simulink model "BEST2020_gamepad_template"  (R2020a)
settings: Solver=ode23t  StartTime=0.0  StopTime=180.1  FixedStep=0.05  RelTol=1e-3  EnableMultiTasking=on
model workspace (MAT data in the model file):
  mapForSim.obsMap = [0 0 0 0 0 0 0 0 0 0 0 0 ... (4194304 elements, 2048x2048)]
  mapForSim.scaleFactor = 409.6
  mapForSim.simMap = robotics.BinaryOccupancyGrid
  mapForSim.simMap.Grid = [1 1 1 1 1 1 1 1 1 1 1 1 ... (4194304 elements, 2048x2048)]
  mapForSim.simMap.LayerName = "binaryLayer"
  mapForSim.simMap.Index = matlabshared.autonomous.internal.CircularBufferIndex
  mapForSim.simMap.Index.Head = [1 1]
  mapForSim.simMap.Index.Size = [2048 2048]
  mapForSim.simMap.Index.NewRegions = [0 0 0 0]
  mapForSim.simMap.Index.DropEntireMap = 0
  mapForSim.simMap.Index.DropTwoRegions = [0 0]
  mapForSim.simMap.Buffer = matlabshared.autonomous.internal.CircularBuffer
  mapForSim.simMap.Buffer.ConstVal = 0
  mapForSim.simMap.Buffer.DataType = 'logical'
  mapForSim.simMap.Buffer.Index = matlabshared.autonomous.internal.CircularBufferIndex
  mapForSim.simMap.Buffer.Index.Head = [1 1]
  mapForSim.simMap.Buffer.Index.Size = [2048 2048]
  mapForSim.simMap.Buffer.Index.NewRegions = [0 0 0 0]
  mapForSim.simMap.Buffer.Index.DropEntireMap = 0
  mapForSim.simMap.Buffer.Index.DropTwoRegions = [0 0]
  mapForSim.simMap.Buffer.Buffer = [1 1 1 1 1 1 1 1 1 1 1 1 ... (4194304 elements, 2048x2048)]
  mapForSim.simMap.DefaultValueInternal = 0
  mapForSim.simMap.HasParent = 0
  mapForSim.simMap.Resolution = 409.6
  mapForSim.simMap.GridSize = [2048 2048]
  mapForSim.simMap.GridOriginInLocal = [0 0]
  mapForSim.simMap.LocalOriginInWorld = [0 0]
  mapForSim.simMap.Width = 5
  mapForSim.simMap.Height = 5
  mapForSim.simMap.LocalOriginInWorldInternal = [0 0]
  occGrid = robotics.BinaryOccupancyGrid
  occGrid.Grid = [1 1 1 1 1 1 1 1 1 1 1 1 ... (4194304 elements, 2048x2048)]
  occGrid.LayerName = "binaryLayer"
  occGrid.Index = matlabshared.autonomous.internal.CircularBufferIndex
  occGrid.Index.Head = [1 1]
  occGrid.Index.Size = [2048 2048]
  occGrid.Index.NewRegions = [0 0 0 0]
  occGrid.Index.DropEntireMap = 0
  occGrid.Index.DropTwoRegions = [0 0]
  occGrid.Buffer = matlabshared.autonomous.internal.CircularBuffer
  occGrid.Buffer.ConstVal = 0
  occGrid.Buffer.DataType = 'logical'
  occGrid.Buffer.Index = matlabshared.autonomous.internal.CircularBufferIndex
  occGrid.Buffer.Index.Head = [1 1]
  occGrid.Buffer.Index.Size = [2048 2048]
  occGrid.Buffer.Index.NewRegions = [0 0 0 0]
  occGrid.Buffer.Index.DropEntireMap = 0
  occGrid.Buffer.Index.DropTwoRegions = [0 0]
  occGrid.Buffer.Buffer = [1 1 1 1 1 1 1 1 1 1 1 1 ... (4194304 elements, 2048x2048)]
  occGrid.DefaultValueInternal = 0
  occGrid.HasParent = 0
  occGrid.Resolution = 409.6
  occGrid.GridSize = [2048 2048]
  occGrid.GridOriginInLocal = [0 0]
  occGrid.LocalOriginInWorld = [0 0]
  occGrid.Width = 5
  occGrid.Height = 5
  occGrid.LocalOriginInWorldInternal = [0 0]
undefined symbols (not defined in the file): cellLevel, cellPose, cellTypeArray, FloorSurface, isoPoses, platformPoses, PlowSurface, Ref, RobotSurface, WallSurface, X, Y, Z
libraries: sm_lib x286, nesl_utility x157, simulink x72, vexcommonlib x2, vrlib x1
(part 1 of 14)
settings Model: EnablePacing=on  ExtModeTrigDuration=25  Creator=scastro  LastModifiedBy=Hashim Aziz
settings SolverCC: AlgebraicLoopSolver=LineSearch
settings DataIOCC: LimitDataPoints=on  ReturnWorkspaceOutputs=off
settings OptimizationCC: DefaultParameterBehavior=Inlined  PassReuseOutputArgsAs=Individual arguments  MaxStackSize=64  EfficientTunableParamExpr=on
settings DebuggingCC: ParameterPrecisionLossMsg=none  ParameterTunabilityLossMsg=error  UnconnectedLineMsg=none  AllowSymbolicDim=off  SFUnexpectedBacktrackingDiag=warning  SFNoUnconditionalDefaultTransitionDiag=warning  SFExecutionAtInitializationDiag=none  ArithmeticOperatorsInVariantConditions=warning
settings HardwareCC: ProdBitPerPointer=32  ProdBitPerSizeT=32  ProdBitPerPtrDiffT=32  ProdLargestAtomicInteger=Long  ProdLargestAtomicFloat=Double  ProdWordSize=32  ProdHWDeviceType=ARM Compatible->ARM Cortex
settings SFSimCC: SimUseLocalCustomCode=off  MATLABDynamicMemAlloc=off  CustomCodeUndefinedFunction=UseInterfaceOnly
settings RTWCC: SystemTargetFile=ert.tlc  TemplateMakefile=ert_default_tmf  GenerateReport=on  RTWUseLocalCustomCode=off  Toolchain=GNU Tools for ARM Embedded Processors  IncludeHyperlinkInReport=on  LaunchReport=on  GenerateTraceInfo=on  GenerateTraceReport=on  GenerateTraceReportSl=on  GenerateTraceReportSf=on  GenerateTraceReportEml=on
settings CodeAppCC: ForceParamTrailComments=on  IgnoreCustomStorageClasses=off  OperatorAnnotations=on  SimulinkDataObjDesc=on  SFDataObjDesc=on  InsertBlockDesc=on
settings ERTTargetCC: ExtModeStaticAllocSize=2048  ERTCustomFileTemplate=example_file_process.tlc
settings ConfigComp: CovMetricSettings=dw  CovHtmlReporting=on  CovSaveCumulativeToWorkspaceVar=on  CovSaveSingleToWorkspaceVar=on  CovExternalEMLEnable=off  CovSFcnEnable=off
settings SimscapeCC: SimscapeNominalValues="[{\"value\":\"10\",\"unit\":\"V\"},{\"value\":\"1\",\"unit\":\"A\"},{\"value\":\"10\",\"unit\":\"N*m\"},{\"value\":\"10\",\"unit\":\"bar\"},{\"value\":\"100\",\"unit\":\"kJ/kg\"},{\"value\":\"1\",\"unit\":\"kW\"},{\"value\":\"300\",\"unit\":\"K\"},{\"value\":\"100\",\"unit\":\"cm^3/s\"},{\"value\":\"1\",\"unit\":\"kN\"},{\"value\":\"1\",\"unit\":\"g/cm^3\"},{\"value\":\"1\",\"unit\":\"l\"},{\"value\":\"1\",\"unit\":\"cm^2\"},{\"value\":\"60\",\"unit\":\"Hz\"}]"  SimscapeLogOpenViewer=on  SimscapeLogDataHistory=10000
settings ConfigurationSet: Description=SimMechanics 2G
settings DiagnosticsConfigSet: SimMechanicsRigidlyBoundBlock=none
settings ExplorerConfigSet: InternalSimMechanicsExplorerSettings="<ExplorerConfiguration><canonicalview>default</canonicalview><AnimationSetting><BasePlaybackSpeed>1.0</BasePlaybackSpeed><PlaybackSpeedFactor>1.0</PlaybackSpeedFactor></AnimationSetting><TilePanel><TileInfo><Tiles Columns=\"2\" Count=\"3\" Rows=\"2\"><Column Weight=\"0.5\"/><Column Weight=\"0.5\"/><Row Weight=\"0.668\"/><Row Weight=\"0.332\"/><Tile Height=\"1\" Width=\"2\" X=\"0\" Y=\"0\"/><Tile Height=\"1\" Width=\"1\" X=\"0\" Y=\"1\"/><Tile Height=\"1\" Width=\"1\" X=\"1\" Y=\"1\"/></Tiles></TileInfo><SceneInfo><SceneViewer><BGColor><R>0.60000002384185791</R><G>0.60000002384185791</G><B>0.60000002384185791</B></BGColor><Camera><DoPerspective>off</DoPerspective><Position><X>2.41066835351507569</X><Y>-4.14908984137515624</Y><Z>3.70193270331160607</Z></Position><Center><X>1.01728519569986009</X><Y>-1.70616544620136401</Y><Z>1.53735654734938021</Z></Center><Up><X>-0.394111566140174063</X><Y>0.473277490849461246</Y><Z>0.787835319143396218</Z></Up><ViewLimDist>1</ViewLimDist><YLim>1.30936523991048004</YLim><XLim>3.19500799558994419</XLim></Camera></SceneViewer><SceneViewer><BGColor><R>0.60000002384185791</R><G>0.60000002384185791</G><B>0.60000002384185791</B></BGColor><Camera><DoPerspective>on</DoPerspective><Position><X>-2.5</X><Y>0</Y><Z>0.469999999999999973</Z></Position><Center><X>-1.56030737921409157</X><Y>0</Y><Z>0.12797985667433126</Z></Center><Up><X>0.342020143325668713</X><Y>0</Y><Z>0.939692620785908428</Z></Up><ViewLimDist>1</ViewLimDist><YLim>0.466307658154998583</YLim><XLim>1.15289562108260379</XLim></Camera></SceneViewer><SceneViewer><BGColor><R>0.60000002384185791</R><G>0.60000002384185791</G><B>0.60000002384185791</B></BGColor><Camera><DoPerspective>off</DoPerspective><Position><X>-0.165662310308284766</X><Y>-0.309058030467383449</Y><Z>7.45210262533490209</Z></Position><Center><X>-0.165662310308284766</X><Y>-0.309058030467383449</Y><Z>0.069999846435872648</Z></Center><Up><X>0</X><Y>1</Y><Z>-0</Z></Up><ViewLimDist>1</ViewLimDist><YLim>2.10368262272791195</YLim><XLim>5.20112942919845711</XLim></Camera></SceneViewer></SceneInfo></TilePanel><MechEditorPanel><Cameras><Camera><Id>Camera1</Id><Value><Name>RobotView</Name><NativeCamera><PositionTrackingFeature>BEST_Robotics_2020_Game_Double_Click.BEST_2020_Robot.Body.RobotCamera.F</PositionTrackingFeature><CenterTrackingFeature>BEST_Robotics_2020_Game_Double_Click.BEST_2020_Robot.Body.RobotCamera.F</CenterTrackingFeature><UpVectorTrackingFeature>BEST_Robotics_2020_Game_Double_Click.BEST_2020_Robot.Body.RobotCamera.F</UpVectorTrackingFeature><CenterTrackingOrigin>off</CenterTrackingOrigin><CenterTrackingDirection>+X</CenterTrackingDirection><UpVectorTrackingDirection>+Z</UpVectorTrackingDirection></NativeCamera></Value></Camera></Cameras><GfxPanelCameraMap><MapElement CameraMLId=\"Camera1\" GfxPanelIndex=\"1\"/></GfxPanelCameraMap><VideoCreator><PlaybackSpeedRatio>1.0</PlaybackSpeedRatio><FrameRate>30</FrameRate><VideoFormat>Motion JPEG AVI</VideoFormat><FrameSize>auto</FrameSize></VideoCreator></MechEditorPanel></ExplorerConfiguration>"

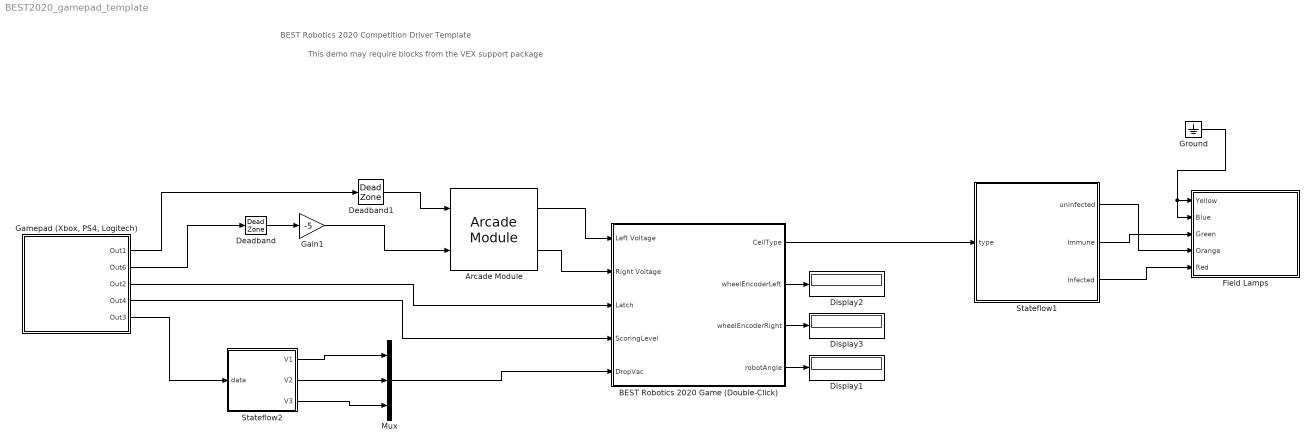
== system BEST2020_gamepad_template ==
  note: BEST Robotics 2020 Competition Driver Template
  note: This demo may require blocks from the VEX support package
  Arcade Module : vexcommonlib/Arcade Module  BlockPlatform=vexarmcortex
      settings: SourceProductBaseCode=EC_VEX_MICRO,VEXV5
  BEST Robotics 2020 Game (Double-Click) : Subsystem  mask(RP BEST Robotics 2020 Challenge){gameTime=180, field=Random, rvis=on, sensor=off, autoField=off, wheelBase=0.5, wheelRadius=0.1, robotColor=[0.5 0 0], wheelThickness=0.025, chassisThickness=0.05, wheelMass=1, chassisMass=1.5}
      mask prompts: gameTime "Game Time (s)"; field "Field Layout"; rvis "Show cell type after run (Runs slower)"; sensor "Activate Gripper Sensor (Not allowed during competition)"; autoField "Autonomous Configuration"; wheelBase "Distance between wheels [m]"; wheelRadius "Wheel radius [m]"; robotColor "Color [R G B]"; wheelThickness "Wheel Thickness [m]"; chassisThickness "Chassis Thickness [m]"; wheelMass "Wheel Mass [kg]"; chassisMass "Chassis Mass [kg]"
      mask help:
      | This block contains a virtual game for the BEST Robotics 2020 competition. Please refere to the instructions provided by competition organizers for more information on game rules.
      |
      | Inputs:
      | Motor Voltages (Torque) [-127 to 127]
      | LatchCell (Pickup Cell) [0 or 1]
      | ScoringLevel (Floor or Platform) [0 or 1]
      | DropVac (Release vaccine) [0 or 1] Array of 3
      |
      | Outputs:
      | Cell Type (Uninfected, Immune, Infected) [0 ,1 or 2]
      | Sensors (See inside block for sensor properties and outputs)
      |
      | For MATLAB and Simulink related questions please email: roboticsarena@mathworks.com
      mask init:
      | autochoice=get_param(gcb,'autoField');
      | choice=get_param(gcb,'field');
      | time=get_param(gcb,'gameTime');
      | set_param(gcs,'StopTime',num2str(str2num(time)+0.1));
      | 
      | if strcmp(choice,'Practice 1')
      |   BEST2020GameConfig1 
      | elseif strcmp(choice,'Practice 2')
      |   BEST2020GameConfig2 
      | elseif strcmp(choice,'Practice 3')
      |   BEST2020GameConfig3 
      | elseif strcmp(choice,'Random')
      |   BEST2020GameConfigRand
      | elseif strcmp(autochoice,"on")
      |    if strcmp(choice,'Competition 1 (Provided during competition)')
      |      BEST2020GameConfigAuto1
      |    elseif strcmp(choice,'Competition 2 (Provided during competition)')
      |      BEST2020GameConfigAuto2
      |    elseif strcmp(choice,'Competition 3 (Provided during competition)')
      |      BEST2020GameConfigAuto3
      |    elseif strcmp(choice,'Competition 4 (Provided during competition)')
      |      BEST2020GameConfigAuto4
      |    elseif strcmp(choice,'Competition 5 (Provided during competition)')
      |      BEST2020GameConfigAuto5
      |    elseif strcmp(choice,'Competition 6 (Provided during competition)')
      |      BEST2020GameConfigAuto6
      |    elseif strcmp(choice,'Competition 7 (Provided during competition)')
      |      BEST2020GameConfigAuto7
      |    elseif strcmp(choice,'Competition 8 (Provided during competition)')
      |      BEST2020GameConfigAuto8
      |    else
      |      BEST2020GameConfigAuto1
      |    end
      | elseif strcmp(choice,'Competition 1 (Provided during competition)')
      |   BEST2020GameConfigComp1
      | elseif strcmp(choice,'Competition 2 (Provided during competition)')
      |   BEST2020GameConfigComp2
      | elseif strcmp(choice,'Competition 3 (Provided during competition)')
      |   BEST2020GameConfigComp3
      | elseif strcmp(choice,'Competition 4 (Provided during competition)')
      |   BEST2020GameConfigComp4
      | elseif strcmp(choice,'Competition 5 (Provided during competition)')
      |   BEST2020GameConfigComp5
      | elseif strcmp(choice,'Competition 6 (Provided during competition)')
      |   BEST2020GameConfigComp6
      | elseif strcmp(choice,'Competition 7 (Provided during competition)')
      |   BEST2020GameConfigComp7
      | elseif strcmp(choice,'Competition 8 (Provided during competition)')
      |   BEST2020GameConfigComp8
      | else
      |   BEST2020GameConfig1 
      | end
      mask TypeOptions field: Practice 1 | Practice 2 | Practice 3 | Random | Competition 1 (Provided during competition) | Competition 2 (Provided during competition) | Competition 3 (Provided during competition) | Competition 4 (Provided during competition) | Competition 5 (Provided during competition) | Competition 6 (Provided during competition) | Competition 7 (Provided during competition) | Competition 8 (Provided during competition)
      mask Callback rvis:
      | visual=get_param(gcb,'rvis');
      | for i=1:21
      |     if strcmp(visual,'off')
      |         set_param([gcb '/Cells/Object' num2str(i) '/EndVisuals'],'Commented','on');
      |     else
      |         set_param([gcb '/Cells/Object' num2str(i) '/EndVisuals'],'Commented','off');
      |     end
      | end
      mask TypeOptions wheelThickness: BEST 2020 Robot/wheelThickness
      mask TypeOptions chassisThickness: BEST 2020 Robot/chassisThickness
      mask TypeOptions wheelMass: BEST 2020 Robot/wheelMass
      mask TypeOptions chassisMass: BEST 2020 Robot/chassisMass
      mask DialogControl Container8 Prompt: Game Settings
      mask DialogControl Container4 Prompt: Robot settings
      mask Display:
      | image('BEST2020Environment.png')
      | port_label('input',1,'RightMotor')
      | port_label('input',2,'LeftMotor')
      | port_label('input',3,'LatchCell')
      | port_label('input',4,'ScoringLevel')
      | port_label('input',5,'DropVac')
      | port_label('output',1,'CellType')
      | port_label('output',2,'LeftEncoder')
      | port_label('output',3,'RightEncoder')
      | port_label('output',4,'RobotAngle')
  Deadband : DeadZone  SaturateOnIntegerOverflow=on
  Deadband1 : DeadZone  SaturateOnIntegerOverflow=on
  Display1 : Display
  Display2 : Display
  Display3 : Display
  Field Lamps : Subsystem
      mask Display:
      | image('lamps.PNG')
      | port_label('input',1,'Yellow')
      | port_label('input',2,'Blue')
      | port_label('input',3,'Green')
      | port_label('input',4,'Orange')
      | port_label('input',5,'Red')
  Gain1 : Gain  Gain=-5
  "Gamepad (Xbox, PS4, Logitech)" : Subsystem
      mask Display:
      | pic = imread(fullfile(codertarget.vexcommon.internal.getRootDir(),'resources','Gamepad_Controller.png'));
      | image(pic);
  Ground : Ground
  Mux : Mux  Inputs=3
  Stateflow1 : Stateflow chart  AncestorBlock=RoboticsPlayground/Utilities and Hardware/Stateflow  TreatAsAtomicUnit=on
  Stateflow2 : Stateflow chart  AncestorBlock=RoboticsPlayground/Utilities and Hardware/Stateflow  TreatAsAtomicUnit=on
  wires:
  Mux/1 -> BEST Robotics 2020 Game (Double-Click)/5(DropVac)
  BEST Robotics 2020 Game (Double-Click)/1(CellType) -> Stateflow1/1(type)
  BEST Robotics 2020 Game (Double-Click)/4(robotAngle) -> Display1/1
  BEST Robotics 2020 Game (Double-Click)/3(wheelEncoderRight) -> Display3/1
  BEST Robotics 2020 Game (Double-Click)/2(wheelEncoderLeft) -> Display2/1
  Arcade Module/1 -> BEST Robotics 2020 Game (Double-Click)/1(Left Voltage)
  Arcade Module/2 -> BEST Robotics 2020 Game (Double-Click)/2(Right Voltage)
  Gain1/1 -> Arcade Module/2
  Deadband/1 -> Gain1/1
  Deadband1/1 -> Arcade Module/1
  "Gamepad (Xbox, PS4, Logitech)"/4(Out4) -> BEST Robotics 2020 Game (Double-Click)/4(ScoringLevel)
  Stateflow1/3(Infected) -> Field Lamps/5(Red)
  Stateflow1/2(Immune) -> Field Lamps/3(Green)
  Stateflow1/1(uninfected) -> Field Lamps/4(Orange)
  Ground/1 -> Field Lamps/2(Blue), Field Lamps/1(Yellow)
  Stateflow2/1(V1) -> Mux/1
  Stateflow2/2(V2) -> Mux/2
  Stateflow2/3(V3) -> Mux/3
  "Gamepad (Xbox, PS4, Logitech)"/5(Out3) -> Stateflow2/1(data)
  "Gamepad (Xbox, PS4, Logitech)"/1(Out1) -> Deadband1/1
  "Gamepad (Xbox, PS4, Logitech)"/2(Out6) -> Deadband/1
  "Gamepad (Xbox, PS4, Logitech)"/3(Out2) -> BEST Robotics 2020 Game (Double-Click)/3(Latch)

== system BEST2020_gamepad_template/BEST Robotics 2020 Game (Double-Click) ==
  note: DO NOT CHANGE THIS MODEL!
  Left Voltage : Inport
  Right Voltage : Inport  Port=2
  Latch : Inport  Port=3
  ScoringLevel : Inport  Port=4
  DropVac : Inport  Port=5
  Arena : Subsystem  mask(RP Grid Arena){length=7, width=7}
      mask prompts: length "Arena length [m]"; width "Arena width [m]"
      mask help: This block is an arena for robots to operate within. This arena implements contact between one robot and the walls and also introduces a floor grid for better visualization. Connect to other robots within the library using the corresponding "Robot" and "Ref" ports.
      mask DialogControl Container5 Prompt: Arena dimensions
      mask Display:
      | image('BEST2020Arena.png')
      | port_label('Lconn',1,'RP-Bus')
  BEST 2020 Robot : Subsystem  mask(RP Contact Tank Robot){robotId=1, wheelRadius=wheelRadius, wheelBase=wheelBase, wheelThickness=wheelThickness, chassisThickness=chassisThickness, startPose=[-2 0], choice=off, sensorTs=0.05, wheelMass=wheelMass, chassisMass=chassisMass, maxWheelTorque=2, wheelColor=[0.25 0.25 0.25], chassisColor=robotColor}
      mask prompts: robotId "Robot ID"; wheelRadius "Wheel Radius [m]"; wheelBase "Wheelbase [m]"; wheelThickness "Wheel Thickness [m]"; chassisThickness "Chassis Thickness [m]"; startPose "Start Position [m]"; choice "Reverse Start Position"; sensorTs "Sensor sample time [s]"; wheelMass "Wheel Mass [kg]"; chassisMass "Chassis Mass [kg]"; maxWheelTorque "Maximum wheel torque [N*m]"; wheelColor "Wheel Color"; chassisColor "Chassis Color"
      mask help:
      | This robot implements contact between the robot wheels and the floor of an arena. The stck-slip friction implemented using contact force libraries makes the robot behavior more realistic. The inputs to the robot are now motor torque, which is set using the Robotics Playground Motor blocks. The motor mappings are as follows:
      |
      | Motor 1 -> Left wheel motor torque
      | Motor 2 -> Right wheel motor torque
      mask DialogControl KinContainer Prompt: Kinematics
      mask DialogControl DynamicsContainer Prompt: Dynamics
      mask DialogControl AppearanceContainer Prompt: Appearance
      mask Display:
      | image('BEST2020Robot.png')
      | port_label('Rconn',1,'RP-Bus')
  Cells : Subsystem
      mask Display: image('BEST2020Cells.png')
  Compass Sensor : Subsystem  mask(RP Compass Sensor){sensorTs=0.1}
      mask prompts: sensorTs "Sensor sample time [s]"
      mask help: This sensor outputs the rotation in degrees as measured from the robot center relative to the world coordinate frame.
      mask Help: web('compass_sensor.htm')
      mask DialogControl senCont Prompt: Sensor Characteristics
      mask Display:
      | color('white');
      | plot([100,100,100,100]*1,[100,100,100,100]*1);
      | plot([100,100,100,100]*0,[100,100,100,100]*0);
      | image('Compass.png','center')
      | color('blue');
  Game Control : Subsystem
  Left Encoder : Subsystem  mask(RP Motor Encoder){rstChoice=No reset, ticks=180, detectDir=off, sensorTs=0.1}
      mask prompts: rstChoice "Reset option"; ticks "Ticks per rotation"; detectDir "Detect direction of rotation"; sensorTs "Sensor sample time [s]"
      mask help:
      | This block outputs the rotation in tick counts of an encoder conneted to the respective robot motor. You can set different sensor parameters from the mask or use the default settings.
      |
      | The most common use of motor encoders is to derive the position of an object. Start by converting the tick counts to revolutions of the motor shaft. You can later relate the revolutions of the motor shaft to more valuable robot information such as traveled distance by using robot dimensions like the wheel size.
      mask Help: web('encoder_sensor.htm')
      mask TypeOptions rstChoice: No reset | Reset by external signal
      mask DialogControl ParameterGroupVar Prompt: Settings
      mask Display:
      | color('white');
      | plot([100,100,100,100]*1,[100,100,100,100]*1);
      | plot([100,100,100,100]*0,[100,100,100,100]*0);
      | image('encoder.jpg','center')
  Right Encoder : Subsystem  mask(RP Motor Encoder){rstChoice=No reset, ticks=180, detectDir=off, sensorTs=0.1}
      mask prompts: rstChoice "Reset option"; ticks "Ticks per rotation"; detectDir "Detect direction of rotation"; sensorTs "Sensor sample time [s]"
      mask help:
      | This block outputs the rotation in tick counts of an encoder conneted to the respective robot motor. You can set different sensor parameters from the mask or use the default settings.
      |
      | The most common use of motor encoders is to derive the position of an object. Start by converting the tick counts to revolutions of the motor shaft. You can later relate the revolutions of the motor shaft to more valuable robot information such as traveled distance by using robot dimensions like the wheel size.
      mask Help: web('encoder_sensor.htm')
      mask TypeOptions rstChoice: No reset | Reset by external signal
      mask DialogControl ParameterGroupVar Prompt: Settings
      mask Display:
      | color('white');
      | plot([100,100,100,100]*1,[100,100,100,100]*1);
      | plot([100,100,100,100]*0,[100,100,100,100]*0);
      | image('encoder.jpg','center')
  Vaccines : Subsystem
      mask Display: image('BEST2020Vaccines.png')
  CellType : Outport
  wheelEncoderLeft : Outport  Port=2
  wheelEncoderRight : Outport  Port=3
  robotAngle : Outport  Port=4
  wires:
  Right Voltage/1 -> BEST 2020 Robot/2(In2)
  Left Voltage/1 -> BEST 2020 Robot/1(In1)
  Latch/1 -> Cells/1(Latch)
  Cells/1(CellType) -> CellType/1
  Right Encoder/1(Out1) -> wheelEncoderRight/1
  Left Encoder/1(Out1) -> wheelEncoderLeft/1
  BEST 2020 Robot/1(leftMotorW) -> Left Encoder/1(In1)
  BEST 2020 Robot/2(rightMotorW) -> Right Encoder/1(In1)
  BEST 2020 Robot/3(angle) -> Compass Sensor/1(angle)
  Compass Sensor/1(Distance) -> robotAngle/1
  DropVac/1 -> Vaccines/2(Drop)
  ScoringLevel/1 -> Vaccines/1("ScoreLevel "), Cells/2(ScoringLevel)
  connections:
  Vaccines/LConn1 -- Arena/LConn1 -- BEST 2020 Robot/RConn1 -- Cells/LConn1

== system BEST2020_gamepad_template/Field Lamps ==
  note: DO NOT EDIT
  note: Inputs should be 0 or 1
  Yellow : Inport
  Blue : Inport  Port=2
  Green : Inport  Port=3
  Orange : Inport  Port=4
  Red : Inport  Port=5
  tag scope: blueLamp=global, greenLamp=global, orangeLamp=global, redLamp=global, yellowLamp=global
  wires:
  Yellow/1 -> [yellowLamp]
  Blue/1 -> [blueLamp]
  Orange/1 -> [orangeLamp]
  Red/1 -> [redLamp]
  Green/1 -> [greenLamp]

== system BEST2020_gamepad_template/Gamepad (Xbox, PS4, Logitech) ==
  note: Use this block for other gamepads
  note: Controller (Logitech or xBox)
  Demux : Demux
  Demux1 : Demux  Outputs=12
  Gamepad Simulator : vexcommonlib/Gamepad Simulator  WhichPad=Logitech Gamepad  JoyId=1  BlockPlatform=vexarmcortex
      settings: SourceProductBaseCode=EC_VEX_MICRO,VEXV5
  Joystick Input : vrlib/Joystick Input  Commented=on  joyid=1  adjustports=on  forcefeed=off
  Rate Transition{1..6,8} (7 alike) : RateTransition  OutPortSampleTime=0.02
  Terminator{1..6,9..13} (11 alike) : Terminator
  Out1 : Outport  VectorParamsAs1DForOutWhenUnconnected=off
  Out6 : Outport  Port=2  VectorParamsAs1DForOutWhenUnconnected=off
  Out2 : Outport  Port=3  VectorParamsAs1DForOutWhenUnconnected=off
  Out4 : Outport  Port=4  VectorParamsAs1DForOutWhenUnconnected=off
  Out3 : Outport  Port=5  VectorParamsAs1DForOutWhenUnconnected=off
  wires:
  Gamepad Simulator/3 -> Rate Transition6/1
  Gamepad Simulator/1 -> Rate Transition3/1
  Gamepad Simulator/16 -> Terminator13/1
  Gamepad Simulator/15 -> Terminator12/1
  Gamepad Simulator/14 -> Terminator11/1
  Gamepad Simulator/13 -> Terminator10/1
  Gamepad Simulator/12 -> Terminator9/1
  Gamepad Simulator/10 -> Rate Transition5/1
  Gamepad Simulator/9 -> Rate Transition4/1
  Gamepad Simulator/8 -> Terminator5/1
  Gamepad Simulator/7 -> Terminator4/1
  Gamepad Simulator/6 -> Terminator3/1
  Gamepad Simulator/5 -> Terminator2/1
  Gamepad Simulator/2 -> Terminator1/1
  Gamepad Simulator/4 -> Rate Transition8/1
  Joystick Input/1 -> Rate Transition1/1
  Joystick Input/2 -> Rate Transition2/1
  Rate Transition1/1 -> Demux/1
  Rate Transition2/1 -> Demux1/1
  Rate Transition3/1 -> Out2/1
  Rate Transition6/1 -> Out1/1
  Rate Transition4/1 -> Out3/1
  Rate Transition5/1 -> Out4/1
  Rate Transition8/1 -> Out6/1
  Gamepad Simulator/11 -> Terminator6/1

== system BEST2020_gamepad_template/BEST Robotics 2020 Game (Double-Click)/Arena ==
  Floor : Subsystem
  Lamps : Subsystem
  Mechanism Configuration : sm_lib/Utilities/Mechanism Configuration  UniformGravity=Constant  GravityVector=[0 0 -9.80665]  GravityUnits=m/s^2  LinearizationDelta=0.001
  Simscape Bus : SimscapeBus  HierarchyStrings=WallSurface;FloorSurface;Ref
  Solver Configuration : nesl_utility/Solver Configuration  PhysicalDomain=network_engine_domain  SubClassName=solver  LeftPortType=input  RightPortType=generic  Tones=[]  Harmonics=[]  SimulateNoise=off  Profile=off  UseLocalSampling=off  EnableSwitchedLinearOptims=on  FrequencyDomain=off  UseCCode=off  RelTol=0.001  AbsTol=1e-06  MinStep=1e-09  ToWorkspace=off  RevertToSquareIcSolve=off  NumHomotopyIterations=100  PhasorMode=off  PhasorModeNumHarmonics=1  DoDC=off  ResidualTolerance=1e-08  UseLocalSolver=off  LocalSolverChoice=NE_BACKWARD_EULER_ADVANCER  LocalSolverSampleTime=0.0002  DoFixedCost=off  MaxNonlinIter=10  MaxModeIter=2  LinearAlgebra=Sparse  EquationFormulation=NE_TIME_EF  DelaysMemoryBudget=1024  AutomaticFiltering=off  FilteringTimeConstant=0.001  PartitionStorageMethod=AS_NEEDED  PartitionMemoryBudget=1024  PartitionMethod=FAST
  World Frame : sm_lib/Frames and Transforms/World Frame
  RP-Bus : PMIOPort  Side=Left
  connections:
  World Frame/RConn1 -- Floor/RConn1 -- Mechanism Configuration/RConn1 -- Simscape Bus/LConn3 -- Lamps/RConn1 -- Solver Configuration/RConn1
  Simscape Bus/RConn1 -- RP-Bus/RConn1
  Simscape Bus/LConn2 -- Floor/LConn1

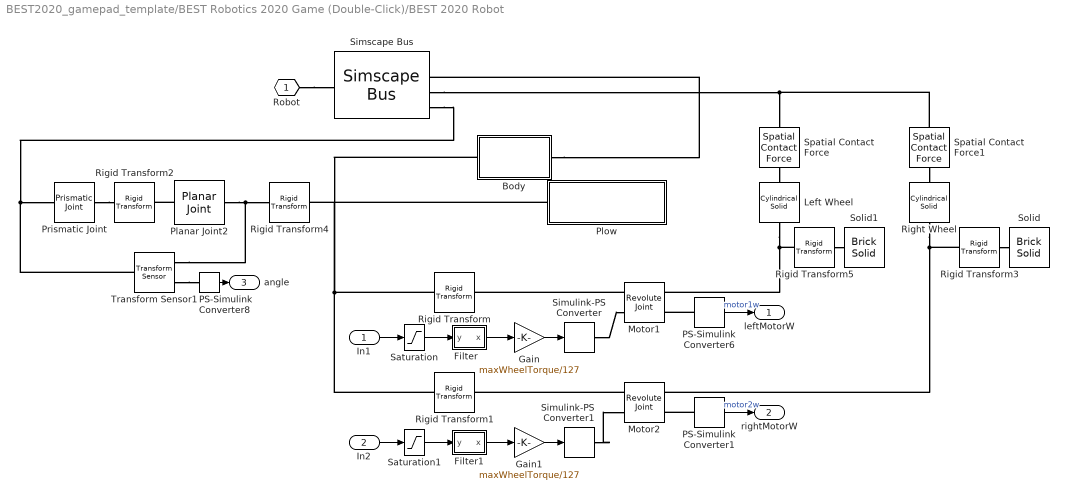
== system BEST2020_gamepad_template/BEST Robotics 2020 Game (Double-Click)/BEST 2020 Robot ==
  In1 : Inport
  In2 : Inport  Port=2
  Body : Subsystem
  Filter : Subsystem
  Filter1 : Subsystem
  Gain : Gain  Gain=maxWheelTorque/127
  Gain1 : Gain  Gain=maxWheelTorque/127
  Left Wheel : sm_lib/Body Elements/Cylindrical Solid  GraphicAmbientColor=[0.15 0.15 0.15 1.0]  BasedOnType=Mass  CenterOfMass=[0 0 0]  CenterOfMassUnits=m  GraphicDiffuseColor=wheelColor  CylinderLength=wheelThickness  CylinderLengthUnits=m  CylinderRadius=wheelRadius  CylinderRadiusUnits=m  Density=1000  DensityUnits=kg/m^3  DoExposeReferenceFrame=on  GraphicEmissiveColor=[0.0 0.0 0.0 1.0]  ExportEntireGeometry=on  SerializedFrames=<Frames/>  MarkerShape=Sphere  MarkerSize=10  GraphicType=FromGeometry  InertiaType=CalculateFromGeometry  Mass=wheelMass  MassUnits=kg  MomentsOfInertia=[1 1 1]  MomentsOfInertiaUnits=kg*m^2  GraphicOpacity=1.0  ProductsOfInertia=[1 1 1]  ProductsOfInertiaUnits=kg*m^2  GraphicShininess=75  GraphicSpecularColor=[0.5 0.5 0.5 1.0]  GraphicVisPropType=SimpleVisualProperties
  Motor1 : sm_lib/Joints/Revolute Joint  JointMode=Normal  SenseConstraintForce=off  SenseConstraintForceX=off  SenseConstraintForceY=off  SenseConstraintForceZ=off  SenseConstraintTorque=off  SenseConstraintTorqueX=off  SenseConstraintTorqueY=off  SenseConstraintTorqueZ=off  SenseTotalForce=off  SenseTotalForceX=off  SenseTotalForceY=off  SenseTotalForceZ=off  SenseTotalTorque=off  SenseTotalTorqueX=off  SenseTotalTorqueY=off  SenseTotalTorqueZ=off  CompositeWrenchDir=FollowerOnBase  CompositeWrenchFrame=BaseFrame  EquilibriumPosition=0  EquilibriumPositionUnits=deg  SpringStiffness=0  SpringStiffnessUnits=N*m/deg  DampingCoefficient=0.004  DampingCoefficientUnits=N*m/(deg/s)  TorqueActuationMode=InputTorque  MotionActuationMode=ComputedMotion  SensePosition=off  SenseVelocity=on  SenseAcceleration=off  SenseTorqueForce=off  SenseLowerLimitTorqueForce=off  SenseUpperLimitTorqueForce=off  LowerLimitSpecify=off  LowerLimitBound=-90  LowerLimitBoundUnits=deg  LowerLimitStiffness=1e4  LowerLimitStiffnessUnits=N*m/deg  LowerLimitDamping=10  LowerLimitDampingUnits=N*m/(deg/s)  LowerLimitTransitionRegionWidth=0.1  LowerLimitTransitionRegionWidthUnits=deg  UpperLimitSpecify=off  UpperLimitBound=90  UpperLimitBoundUnits=deg  UpperLimitStiffness=1e4  UpperLimitStiffnessUnits=N*m/deg  UpperLimitDamping=10  UpperLimitDampingUnits=N*m/(deg/s)  UpperLimitTransitionRegionWidth=0.1  UpperLimitTransitionRegionWidthUnits=deg  PositionTargetSpecify=off  PositionTargetPriority=High  PositionTargetValue=0  PositionTargetValueUnits=deg  VelocityTargetSpecify=off  VelocityTargetPriority=High  VelocityTargetValue=0  VelocityTargetValueUnits=deg/s
  Motor2 : sm_lib/Joints/Revolute Joint  JointMode=Normal  SenseConstraintForce=off  SenseConstraintForceX=off  SenseConstraintForceY=off  SenseConstraintForceZ=off  SenseConstraintTorque=off  SenseConstraintTorqueX=off  SenseConstraintTorqueY=off  SenseConstraintTorqueZ=off  SenseTotalForce=off  SenseTotalForceX=off  SenseTotalForceY=off  SenseTotalForceZ=off  SenseTotalTorque=off  SenseTotalTorqueX=off  SenseTotalTorqueY=off  SenseTotalTorqueZ=off  CompositeWrenchDir=FollowerOnBase  CompositeWrenchFrame=BaseFrame  EquilibriumPosition=0  EquilibriumPositionUnits=deg  SpringStiffness=0  SpringStiffnessUnits=N*m/deg  DampingCoefficient=0.004  DampingCoefficientUnits=N*m/(deg/s)  TorqueActuationMode=InputTorque  MotionActuationMode=ComputedMotion  SensePosition=off  SenseVelocity=on  SenseAcceleration=off  SenseTorqueForce=off  SenseLowerLimitTorqueForce=off  SenseUpperLimitTorqueForce=off  LowerLimitSpecify=off  LowerLimitBound=-90  LowerLimitBoundUnits=deg  LowerLimitStiffness=1e4  LowerLimitStiffnessUnits=N*m/deg  LowerLimitDamping=10  LowerLimitDampingUnits=N*m/(deg/s)  LowerLimitTransitionRegionWidth=0.1  LowerLimitTransitionRegionWidthUnits=deg  UpperLimitSpecify=off  UpperLimitBound=90  UpperLimitBoundUnits=deg  UpperLimitStiffness=1e4  UpperLimitStiffnessUnits=N*m/deg  UpperLimitDamping=10  UpperLimitDampingUnits=N*m/(deg/s)  UpperLimitTransitionRegionWidth=0.1  UpperLimitTransitionRegionWidthUnits=deg  PositionTargetSpecify=off  PositionTargetPriority=High  PositionTargetValue=0  PositionTargetValueUnits=deg  VelocityTargetSpecify=off  VelocityTargetPriority=High  VelocityTargetValue=0  VelocityTargetValueUnits=deg/s
  PS-Simulink Converter1 : nesl_utility/PS-Simulink Converter  PhysicalDomain=network_engine_domain  SubClassName=ps_output  LeftPortType=input  RightPortType=output  PseudoPeriodic=off  Frequencies=[]  Unit=1  AffineConversion=off
  PS-Simulink Converter6 : nesl_utility/PS-Simulink Converter  PhysicalDomain=network_engine_domain  SubClassName=ps_output  LeftPortType=input  RightPortType=output  PseudoPeriodic=off  Frequencies=[]  Unit=1  AffineConversion=off
  PS-Simulink Converter8 : nesl_utility/PS-Simulink Converter  PhysicalDomain=network_engine_domain  SubClassName=ps_output  LeftPortType=input  RightPortType=output  PseudoPeriodic=off  Frequencies=[]  Unit=deg  AffineConversion=off
  Planar Joint2 : sm_lib/Joints/Planar Joint  JointMode=Normal  SenseConstraintForce=off  SenseConstraintForceX=off  SenseConstraintForceY=off  SenseConstraintForceZ=off  SenseConstraintTorque=off  SenseConstraintTorqueX=off  SenseConstraintTorqueY=off  SenseConstraintTorqueZ=off  SenseTotalForce=off  SenseTotalForceX=off  SenseTotalForceY=off  SenseTotalForceZ=off  SenseTotalTorque=off  SenseTotalTorqueX=off  SenseTotalTorqueY=off  SenseTotalTorqueZ=off  CompositeWrenchDir=FollowerOnBase  CompositeWrenchFrame=BaseFrame  PxEquilibriumPosition=0  PxEquilibriumPositionUnits=m  PxSpringStiffness=0  PxSpringStiffnessUnits=N/m  PxDampingCoefficient=0  PxDampingCoefficientUnits=N/(m/s)  PxTorqueActuationMode=NoTorque  PxMotionActuationMode=ComputedMotion  PxSensePosition=off  PxSenseVelocity=off  PxSenseAcceleration=off  PxSenseTorqueForce=off  PxSenseLowerLimitTorqueForce=off  PxSenseUpperLimitTorqueForce=off  PxLowerLimitSpecify=off  PxLowerLimitBound=-1  PxLowerLimitBoundUnits=m  PxLowerLimitStiffness=1e6  PxLowerLimitStiffnessUnits=N/m  PxLowerLimitDamping=1e3  PxLowerLimitDampingUnits=N/(m/s)  PxLowerLimitTransitionRegionWidth=1e-4  PxLowerLimitTransitionRegionWidthUnits=m  PxUpperLimitSpecify=off  PxUpperLimitBound=1  PxUpperLimitBoundUnits=m  PxUpperLimitStiffness=1e6  PxUpperLimitStiffnessUnits=N/m  PxUpperLimitDamping=1e3  PxUpperLimitDampingUnits=N/(m/s)  PxUpperLimitTransitionRegionWidth=1e-4  PxUpperLimitTransitionRegionWidthUnits=m  PxPositionTargetSpecify=on  PxPositionTargetPriority=High  PxPositionTargetValue=startPose(1)  PxPositionTargetValueUnits=m  PxVelocityTargetSpecify=off  PxVelocityTargetPriority=High  PxVelocityTargetValue=0  PxVelocityTargetValueUnits=m/s  PyEquilibriumPosition=0  PyEquilibriumPositionUnits=m  PySpringStiffness=0  PySpringStiffnessUnits=N/m  PyDampingCoefficient=0  PyDampingCoefficientUnits=N/(m/s)  PyTorqueActuationMode=NoTorque  PyMotionActuationMode=ComputedMotion  PySensePosition=off  PySenseVelocity=off  PySenseAcceleration=off  PySenseTorqueForce=off  PySenseLowerLimitTorqueForce=off  PySenseUpperLimitTorqueForce=off  PyLowerLimitSpecify=off  PyLowerLimitBound=-1  PyLowerLimitBoundUnits=m  PyLowerLimitStiffness=1e6  PyLowerLimitStiffnessUnits=N/m  PyLowerLimitDamping=1e3  PyLowerLimitDampingUnits=N/(m/s)  PyLowerLimitTransitionRegionWidth=1e-4  PyLowerLimitTransitionRegionWidthUnits=m  PyUpperLimitSpecify=off  PyUpperLimitBound=1  PyUpperLimitBoundUnits=m  PyUpperLimitStiffness=1e6  PyUpperLimitStiffnessUnits=N/m  PyUpperLimitDamping=1e3  PyUpperLimitDampingUnits=N/(m/s)  PyUpperLimitTransitionRegionWidth=1e-4  PyUpperLimitTransitionRegionWidthUnits=m  PyPositionTargetSpecify=on  PyPositionTargetPriority=High  PyPositionTargetValue=startPose(2)  PyPositionTargetValueUnits=m  PyVelocityTargetSpecify=off  PyVelocityTargetPriority=High  PyVelocityTargetValue=0  PyVelocityTargetValueUnits=m/s  RzEquilibriumPosition=0  RzEquilibriumPositionUnits=deg  RzSpringStiffness=0  RzSpringStiffnessUnits=N*m/deg  RzDampingCoefficient=0  RzDampingCoefficientUnits=N*m/(deg/s)  RzTorqueActuationMode=NoTorque  RzMotionActuationMode=ComputedMotion  RzSensePosition=off  RzSenseVelocity=off  RzSenseAcceleration=off  RzSenseTorqueForce=off  RzSenseLowerLimitTorqueForce=off  RzSenseUpperLimitTorqueForce=off  RzLowerLimitSpecify=off  RzLowerLimitBound=-90  RzLowerLimitBoundUnits=deg  RzLowerLimitStiffness=1e4  RzLowerLimitStiffnessUnits=N*m/deg  RzLowerLimitDamping=10  RzLowerLimitDampingUnits=N*m/(deg/s)  RzLowerLimitTransitionRegionWidth=0.1  RzLowerLimitTransitionRegionWidthUnits=deg  RzUpperLimitSpecify=off  RzUpperLimitBound=90  RzUpperLimitBoundUnits=deg  RzUpperLimitStiffness=1e4  RzUpperLimitStiffnessUnits=N*m/deg  RzUpperLimitDamping=10  RzUpperLimitDampingUnits=N*m/(deg/s)  RzUpperLimitTransitionRegionWidth=0.1  RzUpperLimitTransitionRegionWidthUnits=deg  RzPositionTargetSpecify=off  RzPositionTargetPriority=High  RzPositionTargetValue=0  RzPositionTargetValueUnits=deg  RzVelocityTargetSpecify=off  RzVelocityTargetPriority=High  RzVelocityTargetValue=0  RzVelocityTargetValueUnits=deg/s
  Plow : Subsystem
  Prismatic Joint : sm_lib/Joints/Prismatic Joint  JointMode=Normal  SenseConstraintForce=off  SenseConstraintForceX=off  SenseConstraintForceY=off  SenseConstraintForceZ=off  SenseConstraintTorque=off  SenseConstraintTorqueX=off  SenseConstraintTorqueY=off  SenseConstraintTorqueZ=off  SenseTotalForce=off  SenseTotalForceX=off  SenseTotalForceY=off  SenseTotalForceZ=off  SenseTotalTorque=off  SenseTotalTorqueX=off  SenseTotalTorqueY=off  SenseTotalTorqueZ=off  CompositeWrenchDir=FollowerOnBase  CompositeWrenchFrame=BaseFrame  EquilibriumPosition=0  EquilibriumPositionUnits=m  SpringStiffness=0  SpringStiffnessUnits=N/m  DampingCoefficient=0  DampingCoefficientUnits=N/(m/s)  TorqueActuationMode=NoTorque  MotionActuationMode=ComputedMotion  SensePosition=off  SenseVelocity=off  SenseAcceleration=off  SenseTorqueForce=off  SenseLowerLimitTorqueForce=off  SenseUpperLimitTorqueForce=off  LowerLimitSpecify=off  LowerLimitBound=-1  LowerLimitBoundUnits=m  LowerLimitStiffness=1e6  LowerLimitStiffnessUnits=N/m  LowerLimitDamping=1e3  LowerLimitDampingUnits=N/(m/s)  LowerLimitTransitionRegionWidth=1e-4  LowerLimitTransitionRegionWidthUnits=m  UpperLimitSpecify=off  UpperLimitBound=1  UpperLimitBoundUnits=m  UpperLimitStiffness=1e6  UpperLimitStiffnessUnits=N/m  UpperLimitDamping=1e3  UpperLimitDampingUnits=N/(m/s)  UpperLimitTransitionRegionWidth=1e-4  UpperLimitTransitionRegionWidthUnits=m  PositionTargetSpecify=on  PositionTargetPriority=High  PositionTargetValue=0.02  PositionTargetValueUnits=m  VelocityTargetSpecify=off  VelocityTargetPriority=High  VelocityTargetValue=0  VelocityTargetValueUnits=m/s
  Right Wheel : sm_lib/Body Elements/Cylindrical Solid  GraphicAmbientColor=[0.15 0.15 0.15 1.0]  BasedOnType=Mass  CenterOfMass=[0 0 0]  CenterOfMassUnits=m  GraphicDiffuseColor=wheelColor  CylinderLength=wheelThickness  CylinderLengthUnits=m  CylinderRadius=wheelRadius  CylinderRadiusUnits=m  Density=1000  DensityUnits=kg/m^3  DoExposeReferenceFrame=on  GraphicEmissiveColor=[0.0 0.0 0.0 1.0]  ExportEntireGeometry=on  SerializedFrames=<Frames/>  MarkerShape=Sphere  MarkerSize=10  GraphicType=FromGeometry  InertiaType=CalculateFromGeometry  Mass=wheelMass  MassUnits=kg  MomentsOfInertia=[1 1 1]  MomentsOfInertiaUnits=kg*m^2  GraphicOpacity=1.0  ProductsOfInertia=[1 1 1]  ProductsOfInertiaUnits=kg*m^2  GraphicShininess=75  GraphicSpecularColor=[0.5 0.5 0.5 1.0]  GraphicVisPropType=SimpleVisualProperties
  Rigid Transform : sm_lib/Frames and Transforms/Rigid Transform  TranslationMethod=StandardAxis  TranslationStandardOffset=wheelBase/2  TranslationLengthUnit=m  TranslationStandardAxis=+Y  TranslationCartesianOffset=[0 0 0]  TranslationROffset=0  TranslationROffsetUnits=m  TranslationZOffset=0  TranslationZOffsetUnits=m  TranslationThetaOffset=0  TranslationThetaOffsetUnits=deg  RotationMethod=AlignedAxes  RotationAngleUnits=deg  RotationStandardAxis=+Z  RotationAngle=0.0  RotationArbitraryAxis=[0 0 1]  FollAlignAxisA=+Z  BaseAlignAxisA=+Y  FollAlignAxisB=+X  BaseAlignAxisB=+X  RotationSequenceAxes=FollowerAxes  RotationSequence=XYX  RotationSequenceAngles=[0 0 0]  RotationSequenceAnglesUnits=deg  RotationMatrix=[1 0 0; 0 1 0; 0 0 1]
  Rigid Transform1 : sm_lib/Frames and Transforms/Rigid Transform  TranslationMethod=StandardAxis  TranslationStandardOffset=wheelBase/2  TranslationLengthUnit=m  TranslationStandardAxis=-Y  TranslationCartesianOffset=[0 0 0]  TranslationROffset=0  TranslationROffsetUnits=m  TranslationZOffset=0  TranslationZOffsetUnits=m  TranslationThetaOffset=0  TranslationThetaOffsetUnits=deg  RotationMethod=AlignedAxes  RotationAngleUnits=deg  RotationStandardAxis=+Z  RotationAngle=0.0  RotationArbitraryAxis=[0 0 1]  FollAlignAxisA=+Z  BaseAlignAxisA=+Y  FollAlignAxisB=+X  BaseAlignAxisB=+X  RotationSequenceAxes=FollowerAxes  RotationSequence=XYX  RotationSequenceAngles=[0 0 0]  RotationSequenceAnglesUnits=deg  RotationMatrix=[1 0 0; 0 1 0; 0 0 1]
  Rigid Transform2 : sm_lib/Frames and Transforms/Rigid Transform  TranslationMethod=StandardAxis  TranslationStandardOffset=wheelRadius  TranslationLengthUnit=m  TranslationStandardAxis=+Z  TranslationCartesianOffset=[0 0 0]  TranslationROffset=0  TranslationROffsetUnits=m  TranslationZOffset=0  TranslationZOffsetUnits=m  TranslationThetaOffset=0  TranslationThetaOffsetUnits=deg  RotationMethod=None  RotationAngleUnits=deg  RotationStandardAxis=+Z  RotationAngle=0.0  RotationArbitraryAxis=[0 0 1]  FollAlignAxisA=+Z  BaseAlignAxisA=+Y  FollAlignAxisB=+X  BaseAlignAxisB=+X  RotationSequenceAxes=FollowerAxes  RotationSequence=XYX  RotationSequenceAngles=[0 0 0]  RotationSequenceAnglesUnits=deg  RotationMatrix=[1 0 0; 0 1 0; 0 0 1]
  Rigid Transform3 : sm_lib/Frames and Transforms/Rigid Transform  TranslationMethod=Cartesian  TranslationStandardOffset=0  TranslationLengthUnit=m  TranslationStandardAxis=+Z  TranslationCartesianOffset=[wheelRadius/2 0 0]  TranslationROffset=0  TranslationROffsetUnits=m  TranslationZOffset=0  TranslationZOffsetUnits=m  TranslationThetaOffset=0  TranslationThetaOffsetUnits=deg  RotationMethod=None  RotationAngleUnits=deg  RotationStandardAxis=+Z  RotationAngle=0.0  RotationArbitraryAxis=[0 0 1]  FollAlignAxisA=+X  BaseAlignAxisA=+Y  FollAlignAxisB=+Y  BaseAlignAxisB=+Z  RotationSequenceAxes=FollowerAxes  RotationSequence=XYX  RotationSequenceAngles=[0 0 0]  RotationSequenceAnglesUnits=deg  RotationMatrix=[1 0 0; 0 1 0; 0 0 1]
  Rigid Transform4 : sm_lib/Frames and Transforms/Rigid Transform  TranslationMethod=None  TranslationStandardOffset=0  TranslationLengthUnit=m  TranslationStandardAxis=+Z  TranslationCartesianOffset=[0 0 0]  TranslationROffset=0  TranslationROffsetUnits=m  TranslationZOffset=0  TranslationZOffsetUnits=m  TranslationThetaOffset=0  TranslationThetaOffsetUnits=deg  RotationMethod=StandardAxis  RotationAngleUnits=deg  RotationStandardAxis=+Z  RotationAngle=180*choice  RotationArbitraryAxis=[0 0 1]  FollAlignAxisA=+X  BaseAlignAxisA=+Y  FollAlignAxisB=+Y  BaseAlignAxisB=+Z  RotationSequenceAxes=FollowerAxes  RotationSequence=XYX  RotationSequenceAngles=[0 0 0]  RotationSequenceAnglesUnits=deg  RotationMatrix=[1 0 0; 0 1 0; 0 0 1]
  Rigid Transform5 : sm_lib/Frames and Transforms/Rigid Transform  TranslationMethod=Cartesian  TranslationStandardOffset=0  TranslationLengthUnit=m  TranslationStandardAxis=+Z  TranslationCartesianOffset=[wheelRadius/2 0 0]  TranslationROffset=0  TranslationROffsetUnits=m  TranslationZOffset=0  TranslationZOffsetUnits=m  TranslationThetaOffset=0  TranslationThetaOffsetUnits=deg  RotationMethod=None  RotationAngleUnits=deg  RotationStandardAxis=+Z  RotationAngle=0.0  RotationArbitraryAxis=[0 0 1]  FollAlignAxisA=+X  BaseAlignAxisA=+Y  FollAlignAxisB=+Y  BaseAlignAxisB=+Z  RotationSequenceAxes=FollowerAxes  RotationSequence=XYX  RotationSequenceAngles=[0 0 0]  RotationSequenceAnglesUnits=deg  RotationMatrix=[1 0 0; 0 1 0; 0 0 1]
  Saturation : Saturate  UpperLimit=127  LowerLimit=-127  ZeroCross=off
  Saturation1 : Saturate  UpperLimit=127  LowerLimit=-127  ZeroCross=off
  Simscape Bus : SimscapeBus  HierarchyStrings=PlowSurface;RobotSurface;FloorSurface;Ref
  Simulink-PS Converter : nesl_utility/Simulink-PS Converter  PhysicalDomain=network_engine_domain  SubClassName=ps_input  LeftPortType=input  RightPortType=output  PseudoPeriodic=off  Frequencies=[]  NoiseDistribution=none  NoiseParameters=[]  Unit=1  AffineConversion=off  FilteringAndDerivatives=provide  SimscapeFilterOrder=1  InputFilterTimeConstant=0.05  UdotUserProvided=0
  Simulink-PS Converter1 : nesl_utility/Simulink-PS Converter  PhysicalDomain=network_engine_domain  SubClassName=ps_input  LeftPortType=input  RightPortType=output  PseudoPeriodic=off  Frequencies=[]  NoiseDistribution=none  NoiseParameters=[]  Unit=1  AffineConversion=off  FilteringAndDerivatives=provide  SimscapeFilterOrder=1  InputFilterTimeConstant=0.05  UdotUserProvided=0
  Solid : sm_lib/Body Elements/Brick Solid  GraphicAmbientColor=[0.15 0.15 0.15 1.0]  BasedOnType=Density  BrickDimensions=[wheelRadius*0.8 wheelThickness*1.05 wheelThickness*1.05]  BrickDimensionUnits=m  CenterOfMass=[0 0 0]  CenterOfMassUnits=m  GraphicDiffuseColor=[0.0 0.8 0.8]  Density=1000  DensityUnits=kg/m^3  DoExposeReferenceFrame=on  GraphicEmissiveColor=[0.0 0.0 0.0 1.0]  ExportEntireGeometry=off  SerializedFrames=<Frames/>  MarkerShape=Sphere  MarkerSize=10  GraphicType=FromGeometry  InertiaType=PointMass  Mass=0.001  MassUnits=kg  MomentsOfInertia=[1 1 1]  MomentsOfInertiaUnits=kg*m^2  GraphicOpacity=1.0  ProductsOfInertia=[1 1 1]  ProductsOfInertiaUnits=kg*m^2  GraphicShininess=75  GraphicSpecularColor=[0.5 0.5 0.5 1.0]  GraphicVisPropType=SimpleVisualProperties
  Solid1 : sm_lib/Body Elements/Brick Solid  GraphicAmbientColor=[0.15 0.15 0.15 1.0]  BasedOnType=Density  BrickDimensions=[wheelRadius*0.8 wheelThickness*1.05 wheelThickness*1.05]  BrickDimensionUnits=m  CenterOfMass=[0 0 0]  CenterOfMassUnits=m  GraphicDiffuseColor=[0.0 0.8 0.8]  Density=1000  DensityUnits=kg/m^3  DoExposeReferenceFrame=on  GraphicEmissiveColor=[0.0 0.0 0.0 1.0]  ExportEntireGeometry=off  SerializedFrames=<Frames/>  MarkerShape=Sphere  MarkerSize=10  GraphicType=FromGeometry  InertiaType=PointMass  Mass=0.001  MassUnits=kg  MomentsOfInertia=[1 1 1]  MomentsOfInertiaUnits=kg*m^2  GraphicOpacity=1.0  ProductsOfInertia=[1 1 1]  ProductsOfInertiaUnits=kg*m^2  GraphicShininess=75  GraphicSpecularColor=[0.5 0.5 0.5 1.0]  GraphicVisPropType=SimpleVisualProperties
  Spatial Contact Force : sm_lib/Forces and Torques/Spatial Contact Force  CoefficientOfDynamicFriction=0.5  CoefficientOfStaticFriction=0.7  NormalDamping=1e2  NormalDampingUnits=N/(m/s)  NormalStiffness=1e4  NormalStiffnessUnits=N/m  FrictionalCriticalVelocity=1e-3  FrictionalCriticalVelocityUnits=m/s  ZeroCrossDetectContactStartAndEnd=off  SenseFrictionalForceMagnitude=off  SenseNormalForceMagnitude=off  SenseSeparationDistance=off  NormalTransitionRegionWidth=1e-2  NormalTransitionRegionWidthUnits=m  FrictionType=SmoothStickSlip
  Spatial Contact Force1 : sm_lib/Forces and Torques/Spatial Contact Force  CoefficientOfDynamicFriction=0.5  CoefficientOfStaticFriction=0.7  NormalDamping=1e2  NormalDampingUnits=N/(m/s)  NormalStiffness=1e4  NormalStiffnessUnits=N/m  FrictionalCriticalVelocity=1e-3  FrictionalCriticalVelocityUnits=m/s  ZeroCrossDetectContactStartAndEnd=off  SenseFrictionalForceMagnitude=off  SenseNormalForceMagnitude=off  SenseSeparationDistance=off  NormalTransitionRegionWidth=1e-2  NormalTransitionRegionWidthUnits=m  FrictionType=SmoothStickSlip
  Transform Sensor1 : sm_lib/Frames and Transforms/Transform Sensor  MeasurementFrame=World  SenseAngle=on  SenseAxis=off  SenseAngle1=off  SenseAngle2=off  SenseAngle3=off  SenseQ=off  SenseR=off  SenseOmegaX=off  SenseOmegaY=off  SenseOmegaZ=off  SenseOmega1=off  SenseOmega2=off  SenseOmega3=off  SenseQDot=off  SenseRDot=off  SenseAlphaX=off  SenseAlphaY=off  SenseAlphaZ=off  SenseAlpha1=off  SenseAlpha2=off  SenseAlpha3=off  SenseQDDot=off  SenseRDDot=off  SenseX=off  SenseY=off  SenseZ=off  SenseRad=off  SenseAzim=off  SenseDist=off  SenseInc=off  SenseXDot=off  SenseYDot=off  SenseZDot=off  SenseRadDot=off  SenseAzimDot=off  SenseDistDot=off  SenseIncDot=off  SenseXDDot=off  SenseYDDot=off  SenseZDDot=off  SenseRadDDot=off  SenseAzimDDot=off  SenseDistDDot=off  SenseIncDDot=off
  Robot : PMIOPort  Side=Right
  leftMotorW : Outport
  rightMotorW : Outport  Port=2
  angle : Outport  Port=3
  wires:
  PS-Simulink Converter6/1 -> leftMotorW/1  "motor1w"
  PS-Simulink Converter1/1 -> rightMotorW/1  "motor2w"
  Filter1/1(x) -> Gain1/1
  Filter/1(x) -> Gain/1
  Gain/1 -> Simulink-PS Converter/1
  Gain1/1 -> Simulink-PS Converter1/1
  In1/1 -> Saturation/1
  In2/1 -> Saturation1/1
  PS-Simulink Converter8/1 -> angle/1
  Saturation/1 -> Filter/1(y)
  Saturation1/1 -> Filter1/1(y)
  connections:
  PS-Simulink Converter1/LConn1 -- Motor2/RConn2
  PS-Simulink Converter6/LConn1 -- Motor1/RConn2
  Simulink-PS Converter/RConn1 -- Motor1/LConn2
  Simulink-PS Converter1/RConn1 -- Motor2/LConn2
  Right Wheel/RConn1 -- Rigid Transform3/LConn1 -- Motor2/RConn1
  Motor1/LConn1 -- Rigid Transform/RConn1
  Planar Joint2/LConn1 -- Rigid Transform2/RConn1
  Simscape Bus/LConn4 -- Transform Sensor1/LConn1 -- Prismatic Joint/LConn1
  Motor2/LConn1 -- Rigid Transform1/RConn1
  Rigid Transform5/LConn1 -- Left Wheel/RConn1 -- Motor1/RConn1
  Rigid Transform/LConn1 -- Rigid Transform1/LConn1 -- Body/LConn1 -- Rigid Transform4/RConn1 -- Plow/LConn1
  Planar Joint2/RConn1 -- Rigid Transform4/LConn1 -- Transform Sensor1/RConn1
  Prismatic Joint/RConn1 -- Rigid Transform2/LConn1
  Transform Sensor1/RConn2 -- PS-Simulink Converter8/LConn1
  Robot/RConn1 -- Simscape Bus/RConn1
  Rigid Transform3/RConn1 -- Solid/RConn1
  Rigid Transform5/RConn1 -- Solid1/RConn1
  Spatial Contact Force/RConn1 -- Left Wheel/LConn1
  Spatial Contact Force1/RConn1 -- Right Wheel/LConn1
  Simscape Bus/LConn3 -- Spatial Contact Force1/LConn1 -- Spatial Contact Force/LConn1
  Body/RConn1 -- Simscape Bus/LConn2
